simulink model "Nicholas_DCDC_Boost"  (R2021b)
settings: Solver=VariableStepAuto  StartTime=0.0  StopTime=1e-1  RelTol=1e-3
libraries: spsSeriesRLCBranchLib x3, spsDCVoltageSourceLib x1, spsDiodeLib x1, spsMosfetLib x1, spsMultimeterLib x1, spspowerguiLib x1
settings Model: Creator=NicholasYe  LastModifiedBy=NicholasYe

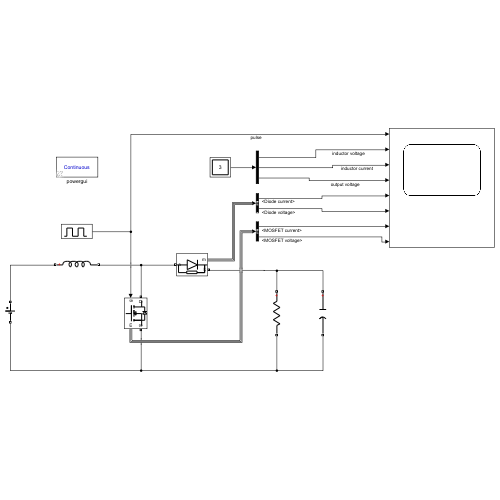
[thumbnail: Simulink's stored preview of the top-level diagram]
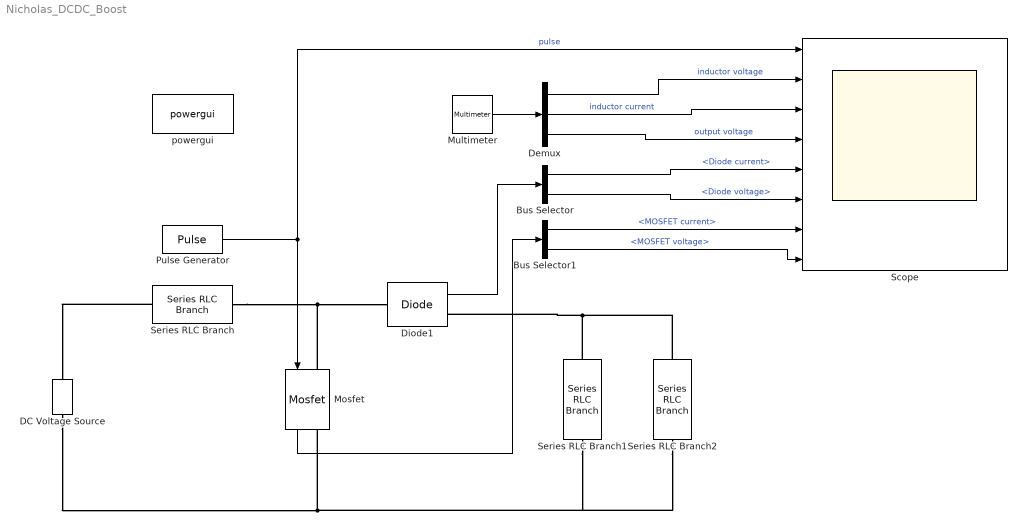
== system Nicholas_DCDC_Boost ==
  Bus Selector : BusSelector  OutputSignals=Diode current,Diode voltage
  Bus Selector1 : BusSelector  OutputSignals=MOSFET current,MOSFET voltage
  DC Voltage Source : spsDCVoltageSourceLib/DC Voltage Source  Amplitude=6  Measurements=None
  Demux : Demux  Outputs=3
  Diode1 : spsDiodeLib/Diode  Ron=0.00000001  Lon=0  Vf=0  IC=0  UseSnubber=0  Rs=500  Cs=250e-9  Measurements=on
  Mosfet : spsMosfetLib/Mosfet  Ron=0.000001  Lon=0  Rd=0.01  Vfd=0  IC=0  Rs=1e5  Cs=inf  Measurements=on
  Multimeter : spsMultimeterLib/Multimeter  PhasorSimulation=off  OutputType=Complex  sel=[1 3 2]  L=3  Gain=[1 1 1]  yselected={'Ub: Series RLC Branch','Ib: Series RLC Branch','Ub: Series RLC Branch1'};  PSBOutputType=1  PSBequivalent=0  AxesSetting=[0,0.1,-100,100]  Display=0  SavedBlockNames=-11
  Pulse Generator : DiscretePulseGenerator  PulseType=Time based  Period=25e-6  PulseWidth=60
  Scope : Scope  NumInputPorts=8
  Series RLC Branch : spsSeriesRLCBranchLib/Series RLC Branch  LConnTagsString=__new0  RConnTagsString=__new0  BranchType=L  Resistance=1  Inductance=12e-6  SetiL0=off  InitialCurrent=0  Capacitance=1e-6  Setx0=off  InitialVoltage=0  Measurements=Branch voltage and current
  Series RLC Branch1 : spsSeriesRLCBranchLib/Series RLC Branch  LConnTagsString=__new0  RConnTagsString=__new0  BranchType=R  Resistance=10  Inductance=1e-3  SetiL0=off  InitialCurrent=0  Capacitance=1e-6  Setx0=off  InitialVoltage=0  Measurements=Branch voltage
  Series RLC Branch2 : spsSeriesRLCBranchLib/Series RLC Branch  LConnTagsString=__new0  RConnTagsString=__new0  BranchType=C  Resistance=1  Inductance=1e-3  SetiL0=off  InitialCurrent=0  Capacitance=1e-3  Setx0=off  InitialVoltage=0  Measurements=None
  powergui : spspowerguiLib/powergui  Priority=1  SimulationMode=Continuous  SampleTime=50e-6  frequency=60  Iterations=50  frequencyindice=0  Pbase=100e6  ErrMax=1e-4  UnitsV=kV  UnitsW=MW  buscounter=0  FunctionMessages=off  echomessages=off  EnableUseOfTLC=off  CurrentSourceSwitches=off  DisableSnubberDevices=off  DisableRonSwitches=off  DisableVfSwitches=off  DisplayEquations=off  AutomaticDiscreteSolvers=off  SolverType=Tustin/Backward Euler (TBE)  Interpol=off  ExternalGateDelay=off  methode=off  Ts=100  x0status=blocks  SPID=on  SwTol=0  HookPort=off  NonlinearTolerance=1e-4  nMaxIteration=100  ContinueOnMaxIteration=off  RestoreLinks=warning  ResistiveCurrentMeasurement=off  Frange=[0:2:500]  Ylog=off  Xlog=on  ShowGrid=off  save=off  variable=ZData  structure=0  ZoomFFT=off  StartTime=0.0  cycles=1  DisplayStyle=1  fundamental=60  FreqAxis=off  MaxFrequency=1000  frequencyindicesteady=1  RmsSteady=1  display=off
  wires:
  Diode1/1 -> Bus Selector/1
  Mosfet/1 -> Bus Selector1/1
  Multimeter/1 -> Demux/1
  Pulse Generator/1 -> Scope/1, Mosfet/1  "pulse"
  Demux/1 -> Scope/2  "inductor voltage"
  Demux/2 -> Scope/3  "inductor current"
  Demux/3 -> Scope/4  "output voltage"
  Bus Selector/1 -> Scope/5  "<Diode current>"
  Bus Selector/2 -> Scope/6  "<Diode voltage>"
  Bus Selector1/1 -> Scope/7  "<MOSFET current>"
  Bus Selector1/2 -> Scope/8  "<MOSFET voltage>"
  connections:
  Series RLC Branch/RConn1 -- Mosfet/LConn1 -- Diode1/LConn1
  Series RLC Branch/LConn1 -- DC Voltage Source/RConn1
  DC Voltage Source/LConn1 -- Series RLC Branch2/RConn1 -- Series RLC Branch1/RConn1 -- Mosfet/RConn1
  Series RLC Branch1/LConn1 -- Diode1/RConn1 -- Series RLC Branch2/LConn1
